simulink model "nonlinear"  (Simulink 6.1)
settings: Solver=ode45  StartTime=0.0  StopTime=60.0  RelTol=1e-3
values from neighbouring files (symbols this model uses):
  b1 = 800    [lin_var.mat]    (also in linear1_param.m = 80; nonlin_var.mat = 400; nonlinear1_param.m = 40)
  b2 = 20    [lin_var.mat]    (also in linear1_param.m; nonlin_var.mat = 10; nonlinear1_param.m = 10)
  fa = 2000    [lin_var.mat]    (also in linear1_param.m; nonlin_var.mat; nonlinear1_param.m)
  k = 600    [lin_var.mat]    (also in linear1_param.m; nonlin_var.mat; nonlinear1_param.m)
  m1 = 70    [lin_var.mat]    (also in linear1_param.m; nonlin_var.mat; nonlinear1_param.m)
  m2 = 500    [lin_var.mat]    (also in linear1_param.m; nonlin_var.mat; nonlinear1_param.m)
settings Model: Creator=m134506  LastModifiedBy=m134506
settings OptimizationCC: InlineInvariantSignals=off  InitFltsAndDblsToZero=off
settings DebuggingCC: SignalResolutionControl=UseLocalSettings  SolverPrmCheckMsg=warning  MultiTaskDSMMsg=error
settings GRTTargetCC: TargetFcnLib=ansi_tfl_table_tmw.mat

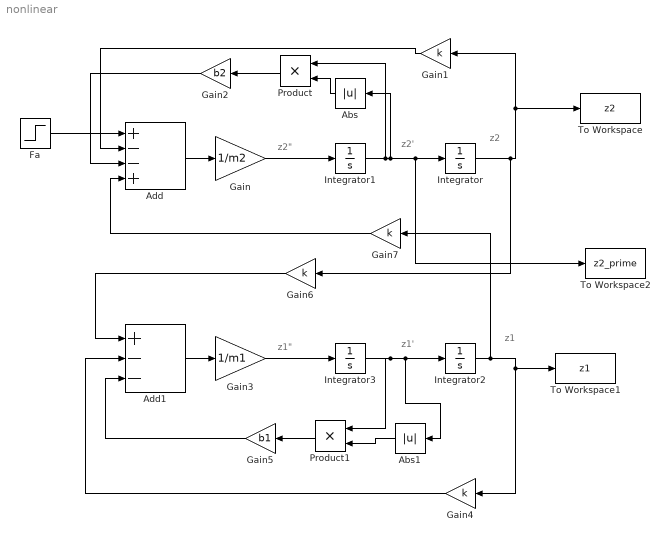
== system nonlinear ==
  note: z2"
  note: z2'
  note: z2
  note: z1"
  note: z1'
  note: z1
  Abs : Abs  Orientation=left
  Abs1 : Abs  Orientation=left
  Add : Sum  Inputs=+--+
  Add1 : Sum  Inputs=+--
  Fa : Step  Time=0  After=fa  SampleTime=0
  Gain : Gain  Gain=1/m2
  Gain{1,4,6..7} (4 alike) : Gain  Orientation=left  Gain=k
  Gain2 : Gain  Orientation=left  Gain=b2
  Gain3 : Gain  Gain=1/m1
  Gain5 : Gain  Orientation=left  Gain=b1
  Integrator{,1..3} (4 alike) : Integrator
  Product : Product  Orientation=left  RndMeth=Zero
  Product1 : Product  Orientation=left  RndMeth=Zero
  To Workspace : ToWorkspace  VariableName=z2  SampleTime=-1  SaveFormat=Array
  To Workspace1 : ToWorkspace  VariableName=z1  SampleTime=-1  SaveFormat=Array
  To Workspace2 : ToWorkspace  VariableName=z2_prime  SampleTime=-1  SaveFormat=Array
  wires:
  Integrator1/1 -> Product/1, Integrator/1, To Workspace2/1, Abs/1
  Gain/1 -> Integrator1/1
  Add/1 -> Gain/1
  Fa/1 -> Add/1
  Integrator/1 -> Gain6/1, Gain1/1, To Workspace/1
  Gain1/1 -> Add/2
  Gain2/1 -> Add/3
  Integrator3/1 -> Product1/1, Integrator2/1, Abs1/1
  Gain3/1 -> Integrator3/1
  Add1/1 -> Gain3/1
  Gain6/1 -> Add1/1
  Integrator2/1 -> Gain7/1, Gain4/1, To Workspace1/1
  Gain4/1 -> Add1/2
  Gain5/1 -> Add1/3
  Gain7/1 -> Add/4
  Product/1 -> Gain2/1
  Product1/1 -> Gain5/1
  Abs/1 -> Product/2
  Abs1/1 -> Product1/2
